simulink model "reglare_cascada"  (R2023a)
settings: Solver=VariableStepAuto  StartTime=0.0  StopTime=2000  RelTol=1e-3
values from neighbouring files (symbols this model uses):
  A = 332.5    [initializare_model.m]
  C = 6.95    [initializare_model.m]
  ho = 17.84    [initializare_model.m]
  hss = 20.61    [initializare_model.m]
  k = 0.033    [initializare_model.m]
  k1 = 0.654    [initializare_model.m]
  k2 = -0.015    [initializare_model.m]
  k3 = -0.0006    [initializare_model.m]
  keta = 8e-5    (= 8e-05)    [initializare_model.m]
  Kp = h/u    (= 1.84666666667)    [initializare_model.m]
  Kp_bucla_interna = 1.13    [initializare_model.m]
  qo = 28.52    [initializare_model.m]
  qss = 34.25    [initializare_model.m]
  Ti_bucla_interna = 13    [initializare_model.m]
  Tp = 0.63 * hss    (= 12.9843)    [initializare_model.m]
libraries: slpidlib x3
settings Model: Creator=evely  LastModifiedBy=evely

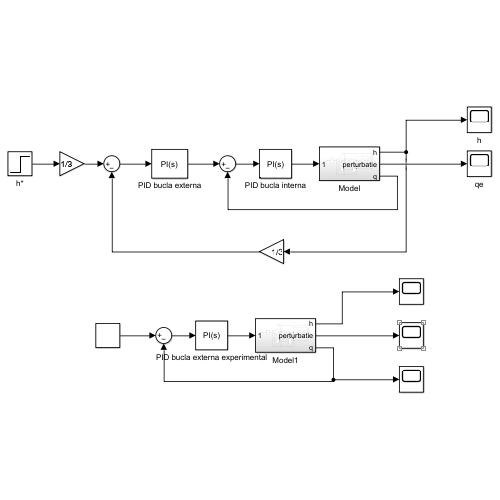
[thumbnail: Simulink's stored preview of the top-level diagram]
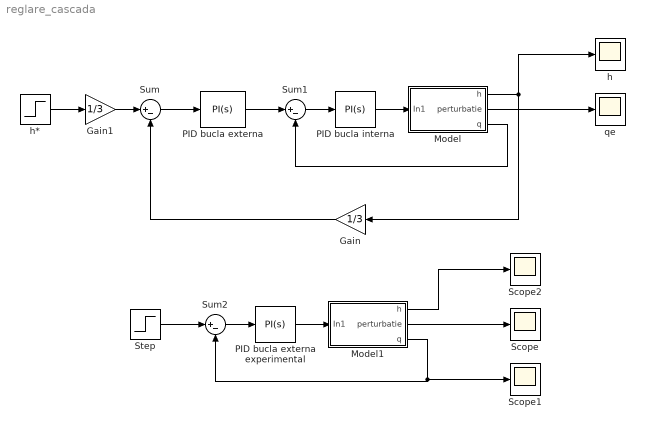
== system reglare_cascada ==
  Gain : Gain  Gain=1/3
  Gain1 : Gain  Gain=1/3
  Model : Subsystem
  Model1 : Subsystem
  PID bucla externa : slpidlib/PID Controller  Controller=PI  Form=Parallel  TimeDomain=Continuous-time  UseExternalTs=off  SampleTime=-1  IntegratorMethod=Forward Euler  FilterMethod=Forward Euler  ControllerParametersSource=internal  P=Kp  I=Kp/Tp  UseKiTs=off  D=0  N=100  UseFilter=on  TunerSelectOption=Transfer Function Based (PID Tuner App)  InitialConditionSource=internal  InitialConditionForIntegrator=uo  InitialConditionForFilter=0  DifferentiatorICPrevScaledInput=0  ExternalReset=none  TrackingMode=off  Kt=1  LimitOutput=off  SatLimitsSource=internal  UpperSaturationLimit=inf  LowerSaturationLimit=-inf  LinearizeAsGain=on  AntiWindupMode=none  Kb=1  LimitIntegrator=off  UpperIntegratorSaturationLimit=inf  LowerIntegratorSaturationLimit=-inf  POutMin=[]  POutMax=[]  IOutMin=[]  IOutMax=[]  DOutMin=[]  DOutMax=[]  NOutMin=[]  NOutMax=[]  SumOutMin=[]  SumOutMax=[]  SaturationOutMin=[]  SaturationOutMax=[]  PParamMin=[]  PParamMax=[]  IParamMin=[]  IParamMax=[]  DParamMin=[]  DParamMax=[]  NParamMin=[]  NParamMax=[]  KbParamMin=[]  KbParamMax=[]  KtParamMin=[]  KtParamMax=[]  KbOutMin=[]  KbOutMax=[]  KtOutMin=[]  KtOutMax=[]  IntegratorOutMin=[]  IntegratorOutMax=[]  FilterOutMin=[]  FilterOutMax=[]  SumI1OutMin=[]  SumI1OutMax=[]  SumI2OutMin=[]  SumI2OutMax=[]  SumI3OutMin=[]  SumI3OutMax=[]  SumI4OutMin=[]  SumI4OutMax=[]  SumDOutMin=[]  SumDOutMax=[]  DifferentiatorOutMin=[]  DifferentiatorOutMax=[]  FilterDiffOutCoefMin=[]  FilterDiffOutCoefMax=[]  ReciprocalOutMin=[]  ReciprocalOutMax=[]  SumDenOutMin=[]  SumDenOutMax=[]  SumNumOutMin=[]  SumNumOutMax=[]  DivideOutMin=[]  DivideOutMax=[]  UdiffTsProdOutMin=[]  UdiffTsProdOutMax=[]  NTsProdOutMin=[]  NTsProdOutMax=[]  UintegralTsProdOutMin=[]  UintegralTsProdOutMax=[]  UngainTsProdOutMin=[]  UngainTsProdOutMax=[]  ClampingZeroOutDataTypeStr=Inherit: Inherit via back propagation  ClampingZeroOutMin=[]  ClampingZeroOutMax=[]  FilterDenConstantOutDataTypeStr=Inherit: Inherit via back propagation  FilterDenConstantOutMin=[]  FilterDenConstantOutMax=[]  PCopyOutDataTypeStr=Inherit: Inherit via back propagation  PCopyOutMin=[]  PCopyOutMax=[]  NCopyOutDataTypeStr=Inherit: Inherit via back propagation  NCopyOutMin=[]  NCopyOutMax=[]  IntegratorContinuousStateAttributes=''  IntegratorStateMustResolveToSignalObject=off  IntegratorRTWStateStorageClass=Auto  FilterContinuousStateAttributes=''  FilterStateMustResolveToSignalObject=off  FilterRTWStateStorageClass=Auto  ParallelPVariant=InternalParameters  IdealPVariant=Disabled  IVariant=InternalParameters  DVariant=Disabled  IntegratorVariant=Continuous  SatVariant=Disabled  AWVariant=Passthrough  PCopyVariant=Disabled  TRVariant=Disabled  FdbkBlocksVariant=Forward  IdealPFdbkVariant=Disabled  SatFdbkVariant=Disabled  DerivativeFilterVariant=Disabled  NVariant=Disabled  NCopyVariant=Disabled_SignalSpec  FilterICVariant=Disabled  IntegratorICVariant=InternalICs  ExternalResetVariant=Disabled  TRSumVariant=Passthrough  SumFdbkVariant=Disabled  SumVariant=Sum_PI  TsampFilterVariant=InternalTs  TsampNgainVariant=Passthrough  TsampIntegralVariant=Disabled_SignalSpec  ExternalSaturationOutDataTypeStr=Inherit: Same as second input
  PID bucla externa experimental : slpidlib/PID Controller  Controller=PI  Form=Parallel  TimeDomain=Continuous-time  UseExternalTs=off  SampleTime=-1  IntegratorMethod=Forward Euler  FilterMethod=Forward Euler  ControllerParametersSource=internal  P=1  I=1  UseKiTs=off  D=0  N=100  UseFilter=on  TunerSelectOption=Transfer Function Based (PID Tuner App)  InitialConditionSource=internal  InitialConditionForIntegrator=0  InitialConditionForFilter=0  DifferentiatorICPrevScaledInput=0  ExternalReset=none  TrackingMode=off  Kt=1  LimitOutput=off  SatLimitsSource=internal  UpperSaturationLimit=inf  LowerSaturationLimit=-inf  LinearizeAsGain=on  AntiWindupMode=none  Kb=1  LimitIntegrator=off  UpperIntegratorSaturationLimit=inf  LowerIntegratorSaturationLimit=-inf  POutMin=[]  POutMax=[]  IOutMin=[]  IOutMax=[]  DOutMin=[]  DOutMax=[]  NOutMin=[]  NOutMax=[]  SumOutMin=[]  SumOutMax=[]  SaturationOutMin=[]  SaturationOutMax=[]  PParamMin=[]  PParamMax=[]  IParamMin=[]  IParamMax=[]  DParamMin=[]  DParamMax=[]  NParamMin=[]  NParamMax=[]  KbParamMin=[]  KbParamMax=[]  KtParamMin=[]  KtParamMax=[]  KbOutMin=[]  KbOutMax=[]  KtOutMin=[]  KtOutMax=[]  IntegratorOutMin=[]  IntegratorOutMax=[]  FilterOutMin=[]  FilterOutMax=[]  SumI1OutMin=[]  SumI1OutMax=[]  SumI2OutMin=[]  SumI2OutMax=[]  SumI3OutMin=[]  SumI3OutMax=[]  SumI4OutMin=[]  SumI4OutMax=[]  SumDOutMin=[]  SumDOutMax=[]  DifferentiatorOutMin=[]  DifferentiatorOutMax=[]  FilterDiffOutCoefMin=[]  FilterDiffOutCoefMax=[]  ReciprocalOutMin=[]  ReciprocalOutMax=[]  SumDenOutMin=[]  SumDenOutMax=[]  SumNumOutMin=[]  SumNumOutMax=[]  DivideOutMin=[]  DivideOutMax=[]  UdiffTsProdOutMin=[]  UdiffTsProdOutMax=[]  NTsProdOutMin=[]  NTsProdOutMax=[]  UintegralTsProdOutMin=[]  UintegralTsProdOutMax=[]  UngainTsProdOutMin=[]  UngainTsProdOutMax=[]  ClampingZeroOutDataTypeStr=Inherit: Inherit via back propagation  ClampingZeroOutMin=[]  ClampingZeroOutMax=[]  FilterDenConstantOutDataTypeStr=Inherit: Inherit via back propagation  FilterDenConstantOutMin=[]  FilterDenConstantOutMax=[]  PCopyOutDataTypeStr=Inherit: Inherit via back propagation  PCopyOutMin=[]  PCopyOutMax=[]  NCopyOutDataTypeStr=Inherit: Inherit via back propagation  NCopyOutMin=[]  NCopyOutMax=[]  IntegratorContinuousStateAttributes=''  IntegratorStateMustResolveToSignalObject=off  IntegratorRTWStateStorageClass=Auto  FilterContinuousStateAttributes=''  FilterStateMustResolveToSignalObject=off  FilterRTWStateStorageClass=Auto  ParallelPVariant=InternalParameters  IdealPVariant=Disabled  IVariant=InternalParameters  DVariant=Disabled  IntegratorVariant=Continuous  SatVariant=Disabled  AWVariant=Passthrough  PCopyVariant=Disabled  TRVariant=Disabled  FdbkBlocksVariant=Forward  IdealPFdbkVariant=Disabled  SatFdbkVariant=Disabled  DerivativeFilterVariant=Disabled  NVariant=Disabled  NCopyVariant=Disabled_SignalSpec  FilterICVariant=Disabled  IntegratorICVariant=InternalICs  ExternalResetVariant=Disabled  TRSumVariant=Passthrough  SumFdbkVariant=Disabled  SumVariant=Sum_PI  TsampFilterVariant=InternalTs  TsampNgainVariant=Passthrough  TsampIntegralVariant=Disabled_SignalSpec  ExternalSaturationOutDataTypeStr=Inherit: Same as second input
  PID bucla interna : slpidlib/PID Controller  Controller=PI  Form=Parallel  TimeDomain=Continuous-time  UseExternalTs=off  SampleTime=-1  IntegratorMethod=Forward Euler  FilterMethod=Forward Euler  ControllerParametersSource=internal  P=Kp_bucla_interna  I=Kp_bucla_interna/Ti_bucla_interna  UseKiTs=off  D=0  N=100  UseFilter=on  TunerSelectOption=Transfer Function Based (PID Tuner App)  InitialConditionSource=internal  InitialConditionForIntegrator=0  InitialConditionForFilter=0  DifferentiatorICPrevScaledInput=0  ExternalReset=none  TrackingMode=off  Kt=1  LimitOutput=off  SatLimitsSource=internal  UpperSaturationLimit=inf  LowerSaturationLimit=-inf  LinearizeAsGain=on  AntiWindupMode=none  Kb=1  LimitIntegrator=off  UpperIntegratorSaturationLimit=inf  LowerIntegratorSaturationLimit=-inf  POutMin=[]  POutMax=[]  IOutMin=[]  IOutMax=[]  DOutMin=[]  DOutMax=[]  NOutMin=[]  NOutMax=[]  SumOutMin=[]  SumOutMax=[]  SaturationOutMin=[]  SaturationOutMax=[]  PParamMin=[]  PParamMax=[]  IParamMin=[]  IParamMax=[]  DParamMin=[]  DParamMax=[]  NParamMin=[]  NParamMax=[]  KbParamMin=[]  KbParamMax=[]  KtParamMin=[]  KtParamMax=[]  KbOutMin=[]  KbOutMax=[]  KtOutMin=[]  KtOutMax=[]  IntegratorOutMin=[]  IntegratorOutMax=[]  FilterOutMin=[]  FilterOutMax=[]  SumI1OutMin=[]  SumI1OutMax=[]  SumI2OutMin=[]  SumI2OutMax=[]  SumI3OutMin=[]  SumI3OutMax=[]  SumI4OutMin=[]  SumI4OutMax=[]  SumDOutMin=[]  SumDOutMax=[]  DifferentiatorOutMin=[]  DifferentiatorOutMax=[]  FilterDiffOutCoefMin=[]  FilterDiffOutCoefMax=[]  ReciprocalOutMin=[]  ReciprocalOutMax=[]  SumDenOutMin=[]  SumDenOutMax=[]  SumNumOutMin=[]  SumNumOutMax=[]  DivideOutMin=[]  DivideOutMax=[]  UdiffTsProdOutMin=[]  UdiffTsProdOutMax=[]  NTsProdOutMin=[]  NTsProdOutMax=[]  UintegralTsProdOutMin=[]  UintegralTsProdOutMax=[]  UngainTsProdOutMin=[]  UngainTsProdOutMax=[]  ClampingZeroOutDataTypeStr=Inherit: Inherit via back propagation  ClampingZeroOutMin=[]  ClampingZeroOutMax=[]  FilterDenConstantOutDataTypeStr=Inherit: Inherit via back propagation  FilterDenConstantOutMin=[]  FilterDenConstantOutMax=[]  PCopyOutDataTypeStr=Inherit: Inherit via back propagation  PCopyOutMin=[]  PCopyOutMax=[]  NCopyOutDataTypeStr=Inherit: Inherit via back propagation  NCopyOutMin=[]  NCopyOutMax=[]  IntegratorContinuousStateAttributes=''  IntegratorStateMustResolveToSignalObject=off  IntegratorRTWStateStorageClass=Auto  FilterContinuousStateAttributes=''  FilterStateMustResolveToSignalObject=off  FilterRTWStateStorageClass=Auto  ParallelPVariant=InternalParameters  IdealPVariant=Disabled  IVariant=InternalParameters  DVariant=Disabled  IntegratorVariant=Continuous  SatVariant=Disabled  AWVariant=Passthrough  PCopyVariant=Disabled  TRVariant=Disabled  FdbkBlocksVariant=Forward  IdealPFdbkVariant=Disabled  SatFdbkVariant=Disabled  DerivativeFilterVariant=Disabled  NVariant=Disabled  NCopyVariant=Disabled_SignalSpec  FilterICVariant=Disabled  IntegratorICVariant=InternalICs  ExternalResetVariant=Disabled  TRSumVariant=Passthrough  SumFdbkVariant=Disabled  SumVariant=Sum_PI  TsampFilterVariant=InternalTs  TsampNgainVariant=Passthrough  TsampIntegralVariant=Disabled_SignalSpec  ExternalSaturationOutDataTypeStr=Inherit: Same as second input
  Scope : Scope
  Scope1 : Scope
  Scope2 : Scope
  Step : Step  Time=0  Before=qo  After=qss  SampleTime=0
  Sum : Sum  Inputs=|+-
  Sum1 : Sum  Inputs=|+-
  Sum2 : Sum  Inputs=|+-
  h : Scope
  h* : Step  Time=0  Before=ho  After=hss  SampleTime=0
  qe : Scope
  wires:
  Model/1(h) -> Gain/1, h/1
  Gain1/1 -> Sum/1
  PID bucla externa/1 -> Sum1/1
  Gain/1 -> Sum/2
  h*/1 -> Gain1/1
  Sum/1 -> PID bucla externa/1
  Model/2(perturbatie) -> qe/1
  Model/3(q) -> Sum1/2
  Sum1/1 -> PID bucla interna/1
  PID bucla interna/1 -> Model/1(In1)
  PID bucla externa experimental/1 -> Model1/1(In1)
  Sum2/1 -> PID bucla externa experimental/1
  Model1/2(perturbatie) -> Scope/1
  Model1/1(h) -> Scope2/1
  Model1/3(q) -> Sum2/2, Scope1/1
  Step/1 -> Sum2/1

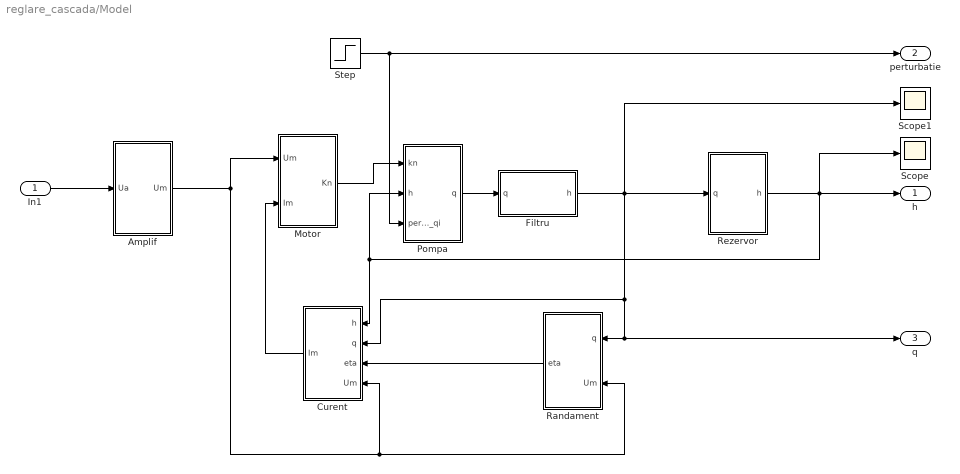
== system reglare_cascada/Model ==
  In1 : Inport
  Amplif : Subsystem
  Curent : Subsystem
  Filtru : Subsystem
  Motor : Subsystem
  Pompa : Subsystem
  Randament : Subsystem
  Rezervor : Subsystem
  Scope : Scope
  Scope1 : Scope
  Step : Step  Time=750  After=0.01  SampleTime=0
  h : Outport
  perturbatie : Outport  Port=2
  q : Outport  Port=3
  wires:
  In1/1 -> Amplif/1(Ua)
  Filtru/1(h) -> Scope1/1, Rezervor/1(q), q/1, Randament/1(q), Curent/2(q)
  Rezervor/1(h) -> Scope/1, h/1, Curent/1(h), Pompa/2(h)
  Amplif/1(Um) -> Motor/1(Um), Randament/2(Um), Curent/4(Um)
  Randament/1(eta) -> Curent/3(eta)
  Curent/1(Im) -> Motor/2(Im)
  Pompa/1(q) -> Filtru/1(q)
  Motor/1(Kn) -> Pompa/1(kn)
  Step/1 -> Pompa/3(perturbatie_qi), perturbatie/1

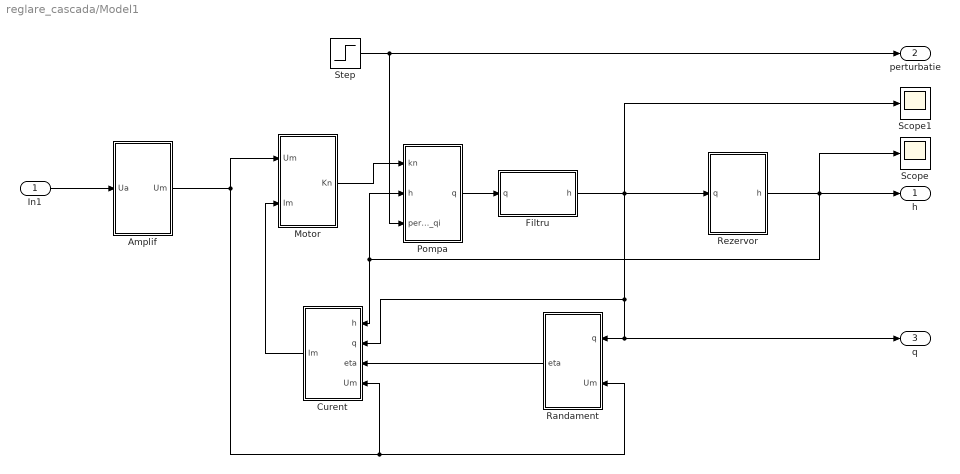
== system reglare_cascada/Model1 ==
  In1 : Inport
  Amplif : Subsystem
  Curent : Subsystem
  Filtru : Subsystem
  Motor : Subsystem
  Pompa : Subsystem
  Randament : Subsystem
  Rezervor : Subsystem
  Scope : Scope
  Scope1 : Scope
  Step : Step  Time=750  After=0.01  SampleTime=0
  h : Outport
  perturbatie : Outport  Port=2
  q : Outport  Port=3
  wires:
  In1/1 -> Amplif/1(Ua)
  Filtru/1(h) -> Scope1/1, Rezervor/1(q), q/1, Randament/1(q), Curent/2(q)
  Rezervor/1(h) -> Scope/1, h/1, Curent/1(h), Pompa/2(h)
  Amplif/1(Um) -> Motor/1(Um), Randament/2(Um), Curent/4(Um)
  Randament/1(eta) -> Curent/3(eta)
  Curent/1(Im) -> Motor/2(Im)
  Pompa/1(q) -> Filtru/1(q)
  Motor/1(Kn) -> Pompa/1(kn)
  Step/1 -> Pompa/3(perturbatie_qi), perturbatie/1

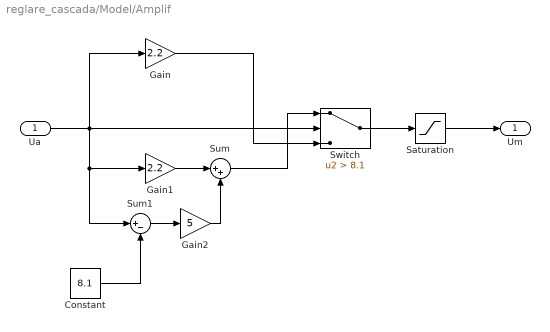
== system reglare_cascada/Model/Amplif ==
  Ua : Inport
  Constant : Constant  Value=8.1
  Gain : Gain  Gain=2.2
  Gain1 : Gain  Gain=2.2
  Gain2 : Gain  Gain=5
  Saturation : Saturate  UpperLimit=22  LowerLimit=0
  Sum : Sum  Inputs=|++
  Sum1 : Sum  Inputs=|+-
  Switch : Switch  Criteria=u2 > Threshold  Threshold=8.1  SaturateOnIntegerOverflow=off  InputSameDT=off
  Um : Outport
  wires:
  Ua/1 -> Gain1/1, Sum1/1, Gain/1, Switch/2
  Gain/1 -> Switch/3
  Switch/1 -> Saturation/1
  Gain1/1 -> Sum/1
  Constant/1 -> Sum1/2
  Sum1/1 -> Gain2/1
  Gain2/1 -> Sum/2
  Sum/1 -> Switch/1
  Saturation/1 -> Um/1

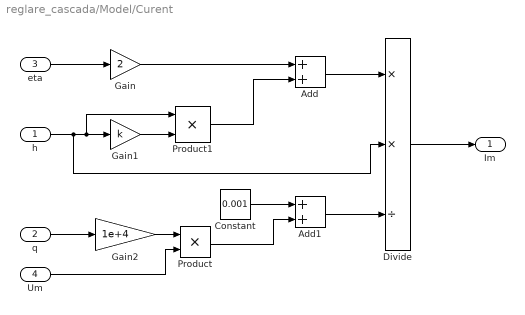
== system reglare_cascada/Model/Curent ==
  h : Inport
  q : Inport  Port=2
  eta : Inport  Port=3
  Um : Inport  Port=4
  Add : Sum
  Add1 : Sum
  Constant : Constant  Value=0.001
  Divide : Product  Inputs=**/
  Gain : Gain  Gain=2
  Gain1 : Gain  Gain=k
  Gain2 : Gain  Gain=1e+4
  Product : Product
  Product1 : Product
  Im : Outport
  wires:
  eta/1 -> Gain/1
  Gain/1 -> Add/1
  h/1 -> Divide/2, Product1/1, Gain1/1
  Gain1/1 -> Product1/2
  Add/1 -> Divide/1
  Product1/1 -> Add/2
  Divide/1 -> Im/1
  q/1 -> Gain2/1
  Gain2/1 -> Product/1
  Um/1 -> Product/2
  Constant/1 -> Add1/1
  Product/1 -> Add1/2
  Add1/1 -> Divide/3

== system reglare_cascada/Model/Filtru ==
  q : Inport
  Integrator : Integrator  InitialCondition=qo
  Sum : Sum  Inputs=|+-
  h : Outport
  wires:
  Sum/1 -> Integrator/1
  Integrator/1 -> Sum/2, h/1
  q/1 -> Sum/1

== system reglare_cascada/Model/Motor ==
  Um : Inport
  Im : Inport  Port=2
  Add : Sum  Inputs=+-
  Rm : Gain  Gain=3
  Kn : Outport
  wires:
  Im/1 -> Rm/1
  Rm/1 -> Add/2
  Um/1 -> Add/1
  Add/1 -> Kn/1

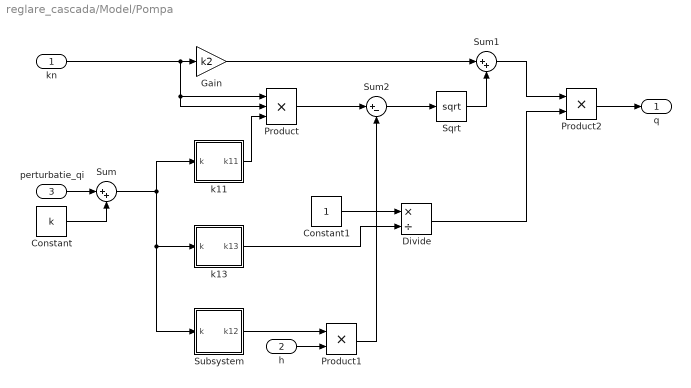
== system reglare_cascada/Model/Pompa ==
  kn : Inport
  h : Inport  Port=2
  perturbatie_qi : Inport  Port=3
  Constant : Constant  Value=k
  Constant1 : Constant
  Divide : Product  Inputs=*/
  Gain : Gain  Gain=k2
  Product : Product  Inputs=3
  Product1 : Product
  Product2 : Product
  Sqrt : Sqrt
  Subsystem : Subsystem
  Sum : Sum  Inputs=|++
  Sum1 : Sum  Inputs=|++
  Sum2 : Sum  Inputs=|+-
  k11 : Subsystem
  k13 : Subsystem
  q : Outport
  wires:
  k11/1(k11) -> Product/3
  Sum2/1 -> Sqrt/1
  k13/1(k13) -> Divide/2
  Divide/1 -> Product2/2
  Sum1/1 -> Product2/1
  Sqrt/1 -> Sum1/2
  perturbatie_qi/1 -> Sum/1
  Constant1/1 -> Divide/1
  Sum/1 -> k11/1(k), Subsystem/1(k), k13/1(k)
  Product2/1 -> q/1
  Subsystem/1(k12) -> Product1/1
  Product/1 -> Sum2/1
  Constant/1 -> Sum/2
  h/1 -> Product1/2
  Product1/1 -> Sum2/2
  kn/1 -> Product/2, Product/1, Gain/1
  Gain/1 -> Sum1/1

== system reglare_cascada/Model/Randament ==
  q : Inport
  Um : Inport  Port=2
  Gain : Gain  Gain=keta
  Product : Product
  eta : Outport
  wires:
  q/1 -> Product/1
  Product/1 -> eta/1
  Um/1 -> Gain/1
  Gain/1 -> Product/2

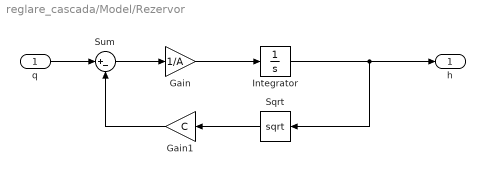
== system reglare_cascada/Model/Rezervor ==
  q : Inport
  Gain : Gain  Gain=1/A
  Gain1 : Gain  Gain=C
  Integrator : Integrator  InitialCondition=ho
  Sqrt : Sqrt
  Sum : Sum  Inputs=|+-
  h : Outport
  wires:
  Integrator/1 -> h/1, Sqrt/1
  Gain/1 -> Integrator/1
  Sum/1 -> Gain/1
  q/1 -> Sum/1
  Sqrt/1 -> Gain1/1
  Gain1/1 -> Sum/2

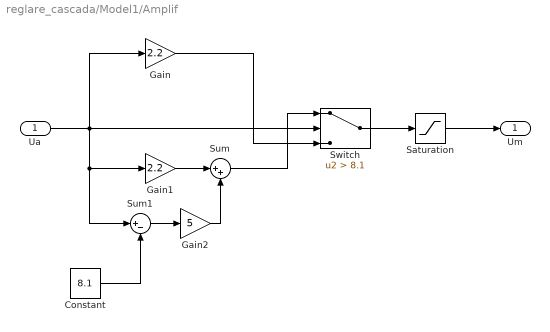
== system reglare_cascada/Model1/Amplif ==
  Ua : Inport
  Constant : Constant  Value=8.1
  Gain : Gain  Gain=2.2
  Gain1 : Gain  Gain=2.2
  Gain2 : Gain  Gain=5
  Saturation : Saturate  UpperLimit=22  LowerLimit=0
  Sum : Sum  Inputs=|++
  Sum1 : Sum  Inputs=|+-
  Switch : Switch  Criteria=u2 > Threshold  Threshold=8.1  SaturateOnIntegerOverflow=off  InputSameDT=off
  Um : Outport
  wires:
  Ua/1 -> Gain1/1, Sum1/1, Gain/1, Switch/2
  Gain/1 -> Switch/3
  Switch/1 -> Saturation/1
  Gain1/1 -> Sum/1
  Constant/1 -> Sum1/2
  Sum1/1 -> Gain2/1
  Gain2/1 -> Sum/2
  Sum/1 -> Switch/1
  Saturation/1 -> Um/1

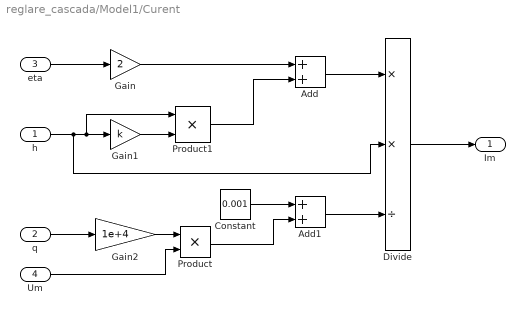
== system reglare_cascada/Model1/Curent ==
  h : Inport
  q : Inport  Port=2
  eta : Inport  Port=3
  Um : Inport  Port=4
  Add : Sum
  Add1 : Sum
  Constant : Constant  Value=0.001
  Divide : Product  Inputs=**/
  Gain : Gain  Gain=2
  Gain1 : Gain  Gain=k
  Gain2 : Gain  Gain=1e+4
  Product : Product
  Product1 : Product
  Im : Outport
  wires:
  eta/1 -> Gain/1
  Gain/1 -> Add/1
  h/1 -> Divide/2, Product1/1, Gain1/1
  Gain1/1 -> Product1/2
  Add/1 -> Divide/1
  Product1/1 -> Add/2
  Divide/1 -> Im/1
  q/1 -> Gain2/1
  Gain2/1 -> Product/1
  Um/1 -> Product/2
  Constant/1 -> Add1/1
  Product/1 -> Add1/2
  Add1/1 -> Divide/3

== system reglare_cascada/Model1/Filtru ==
  q : Inport
  Integrator : Integrator  InitialCondition=qo
  Sum : Sum  Inputs=|+-
  h : Outport
  wires:
  Sum/1 -> Integrator/1
  Integrator/1 -> Sum/2, h/1
  q/1 -> Sum/1

== system reglare_cascada/Model1/Motor ==
  Um : Inport
  Im : Inport  Port=2
  Add : Sum  Inputs=+-
  Rm : Gain  Gain=3
  Kn : Outport
  wires:
  Im/1 -> Rm/1
  Rm/1 -> Add/2
  Um/1 -> Add/1
  Add/1 -> Kn/1

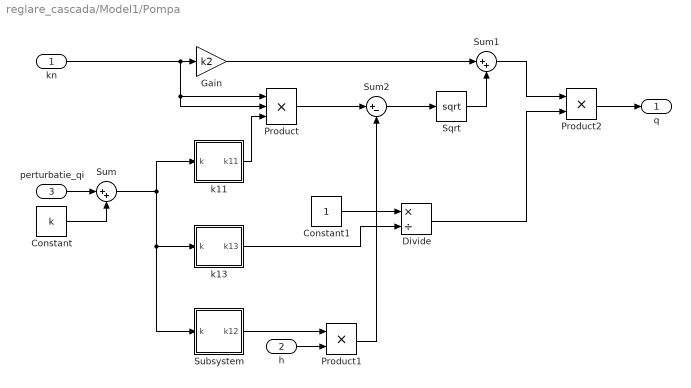
== system reglare_cascada/Model1/Pompa ==
  kn : Inport
  h : Inport  Port=2
  perturbatie_qi : Inport  Port=3
  Constant : Constant  Value=k
  Constant1 : Constant
  Divide : Product  Inputs=*/
  Gain : Gain  Gain=k2
  Product : Product  Inputs=3
  Product1 : Product
  Product2 : Product
  Sqrt : Sqrt
  Subsystem : Subsystem
  Sum : Sum  Inputs=|++
  Sum1 : Sum  Inputs=|++
  Sum2 : Sum  Inputs=|+-
  k11 : Subsystem
  k13 : Subsystem
  q : Outport
  wires:
  k11/1(k11) -> Product/3
  Sum2/1 -> Sqrt/1
  k13/1(k13) -> Divide/2
  Divide/1 -> Product2/2
  Sum1/1 -> Product2/1
  Sqrt/1 -> Sum1/2
  perturbatie_qi/1 -> Sum/1
  Constant1/1 -> Divide/1
  Sum/1 -> k11/1(k), Subsystem/1(k), k13/1(k)
  Product2/1 -> q/1
  Subsystem/1(k12) -> Product1/1
  Product/1 -> Sum2/1
  Constant/1 -> Sum/2
  h/1 -> Product1/2
  Product1/1 -> Sum2/2
  kn/1 -> Product/2, Product/1, Gain/1
  Gain/1 -> Sum1/1

== system reglare_cascada/Model1/Randament ==
  q : Inport
  Um : Inport  Port=2
  Gain : Gain  Gain=keta
  Product : Product
  eta : Outport
  wires:
  q/1 -> Product/1
  Product/1 -> eta/1
  Um/1 -> Gain/1
  Gain/1 -> Product/2

== system reglare_cascada/Model1/Rezervor ==
  q : Inport
  Gain : Gain  Gain=1/A
  Gain1 : Gain  Gain=C
  Integrator : Integrator  InitialCondition=ho
  Sqrt : Sqrt
  Sum : Sum  Inputs=|+-
  h : Outport
  wires:
  Integrator/1 -> h/1, Sqrt/1
  Gain/1 -> Integrator/1
  Sum/1 -> Gain/1
  q/1 -> Sum/1
  Sqrt/1 -> Gain1/1
  Gain1/1 -> Sum/2

== system reglare_cascada/Model/Pompa/Subsystem ==
  k : Inport
  Constant : Constant  Value=k3
  Gain : Gain  Gain=8
  Sum : Sum  Inputs=|+-
  k12 : Outport
  wires:
  k/1 -> Sum/1
  Constant/1 -> Sum/2
  Sum/1 -> Gain/1
  Gain/1 -> k12/1

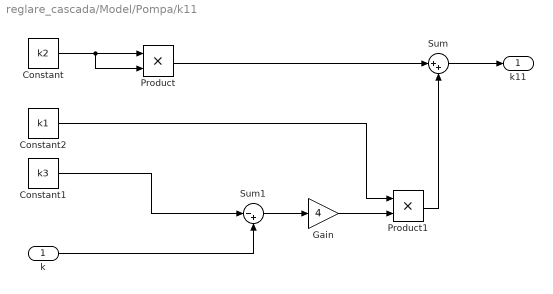
== system reglare_cascada/Model/Pompa/k11 ==
  k : Inport
  Constant : Constant  Value=k2
  Constant1 : Constant  Value=k3
  Constant2 : Constant  Value=k1
  Gain : Gain  Gain=4
  Product : Product
  Product1 : Product
  Sum : Sum  Inputs=|++
  Sum1 : Sum  Inputs=|-+
  k11 : Outport
  wires:
  Constant/1 -> Product/2, Product/1
  Product/1 -> Sum/1
  Constant1/1 -> Sum1/1
  k/1 -> Sum1/2
  Sum1/1 -> Gain/1
  Gain/1 -> Product1/2
  Constant2/1 -> Product1/1
  Product1/1 -> Sum/2
  Sum/1 -> k11/1

== system reglare_cascada/Model/Pompa/k13 ==
  k : Inport
  Constant : Constant  Value=k3
  Gain : Gain  Gain=2
  Sum : Sum  Inputs=|+-
  k13 : Outport
  wires:
  k/1 -> Sum/1
  Constant/1 -> Sum/2
  Sum/1 -> Gain/1
  Gain/1 -> k13/1

== system reglare_cascada/Model1/Pompa/Subsystem ==
  k : Inport
  Constant : Constant  Value=k3
  Gain : Gain  Gain=8
  Sum : Sum  Inputs=|+-
  k12 : Outport
  wires:
  k/1 -> Sum/1
  Constant/1 -> Sum/2
  Sum/1 -> Gain/1
  Gain/1 -> k12/1

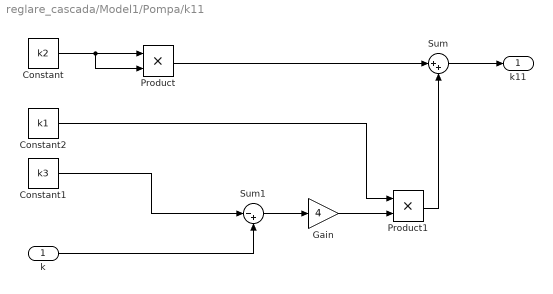
== system reglare_cascada/Model1/Pompa/k11 ==
  k : Inport
  Constant : Constant  Value=k2
  Constant1 : Constant  Value=k3
  Constant2 : Constant  Value=k1
  Gain : Gain  Gain=4
  Product : Product
  Product1 : Product
  Sum : Sum  Inputs=|++
  Sum1 : Sum  Inputs=|-+
  k11 : Outport
  wires:
  Constant/1 -> Product/2, Product/1
  Product/1 -> Sum/1
  Constant1/1 -> Sum1/1
  k/1 -> Sum1/2
  Sum1/1 -> Gain/1
  Gain/1 -> Product1/2
  Constant2/1 -> Product1/1
  Product1/1 -> Sum/2
  Sum/1 -> k11/1

== system reglare_cascada/Model1/Pompa/k13 ==
  k : Inport
  Constant : Constant  Value=k3
  Gain : Gain  Gain=2
  Sum : Sum  Inputs=|+-
  k13 : Outport
  wires:
  k/1 -> Sum/1
  Constant/1 -> Sum/2
  Sum/1 -> Gain/1
  Gain/1 -> k13/1
